simulink model "vendingmachine"  (R2020b)
settings: Solver=VariableStepAuto  StartTime=0.0  StopTime=10.0  RelTol=1e-3
settings Model: Creator=Abhinav dixit  LastModifiedBy=Abhinav dixit

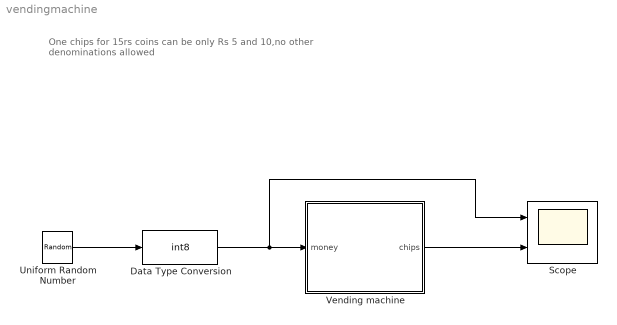
== system vendingmachine ==
  note: One chips for 15rs
      | coins can be only Rs 5 and 10,no other denominations allowed
  Data Type Conversion : DataTypeConversion  OutDataTypeStr=int8  RndMeth=Nearest  SaturateOnIntegerOverflow=on
  Scope : Scope  NumInputPorts=2
  Uniform Random Number : UniformRandomNumber  Minimum=0  Maximum=2  Seed=337  SampleTime=10
  Vending machine : Stateflow chart  TreatAsAtomicUnit=on
  wires:
  Data Type Conversion/1 -> Scope/1, Vending machine/1(money)
  Uniform Random Number/1 -> Data Type Conversion/1
  Vending machine/1(chips) -> Scope/2

== stateflow chart vendingmachine/Vending machine ==
  settings: stateMachineType=MEALY_MACHINE  initializeOutput=1
  state Input_5
  state start
  state Input_10
  (default) -> start
  start -> Input_5 [order 1] : [money==1]{chips=0}
  Input_5 -> start [order 2] : [money==2]{chips=1}
  Input_10 -> start [order 1] : [money==1]{chips=1}
  start -> Input_10 [order 2] : [money==2]{chips=0}
  Input_5 -> Input_10 [order 1] : [money==1]{chips=0}
  Input_10 -> Input_5 [order 2] : [money==2]{chips=1}
  data: money input; chips output
